simulink model "control_system"  (R2020b)
settings: Solver=FixedStepAuto  StartTime=0.0  StopTime=t_sim  FixedStep=Ts  RelTol=1e-2
values from neighbouring files (symbols this model uses):
  Hp = 10    [main_script.m]
  InitPosX = -2.4980e+03    (= -2498)    [main_script.m]
  InitPosY = -650.5503    [main_script.m]
  InitVelX = V0*cosd(InitYaw)    [main_script.m]
  InitVelY = V0*sind(InitYaw)    [main_script.m]
  InitYaw = 21    [main_script.m]
  lr = 1.592    [main_script.m]
  m = 1625    [main_script.m]
  Ts = 0.1    [main_script.m]
  V0 = 25    [main_script.m]
libraries: neural x856, simulink x1, autolibshared x1, drivingscenarioandsensors x1
(part 16 of 40)

== system control_system/50 30 1+2+3+14+15+19 ok curva sx1/Layer 3/Delays 1 ==
  "p{3}" : Inport  PortDimensions=30  SampleTime=0.1
      mask Display: e = 0.06;c1 = [120 230 180]/255;c2 = ([120 230 180]+0)/(256+128);c3 = ([120 230 180]+128)/(256+128);patch([0 1 1 0],[0 0 1 1],c1);patch([0 1 1 1-e 1-e 0+e],[0 0 1 1-e 0+e 0+e],c2);patch([0 0 1 1-e 0+e 0+e],[0 1 1 1-e 1-e 0+e],c3);plot([0 1 1 0 0],[0 0 1 1 0]);
  mux : Mux  Inputs=1
      mask Display: e = 0.06;c1 = [120 150 230]/255;c2 = ([120 150 230]+0)/383;c3 = ([120 150 230]+128)/383;patch([0 1 1 0],[0 0 1 1],c1);patch([0 1 1 1-e 1-e 0+e],[0 0 1 1-e 0+e 0+e],c2);patch([0 0 1 1-e 0+e 0+e],[0 1 1 1-e 1-e 0+e],c3);plot([0 1 1 0 0],[0 0 1 1 0]);disp('Mux')
  "pd{3,2}" : Outport
      mask Display: e = 0.06;c1 = [120 230 180]/255;c2 = ([120 230 180]+0)/(256+128);c3 = ([120 230 180]+128)/(256+128);patch([0 1 1 0],[0 0 1 1],c1);patch([0 1 1 1-e 1-e 0+e],[0 0 1 1-e 0+e 0+e],c2);patch([0 0 1 1-e 0+e 0+e],[0 1 1 1-e 1-e 0+e],c3);plot([0 1 1 0 0],[0 0 1 1 0]);
  wires:
  "p{3}"/1 -> mux/1
  mux/1 -> "pd{3,2}"/1

== system control_system/50 30 1+2+3+14+15+19 ok curva sx1/Layer 3/LW{3,2} ==
  "ad{3,2}" : Inport  PortDimensions=30  SampleTime=0.1
      mask Display: e = 0.06;c1 = [120 230 180]/255;c2 = ([120 230 180]+0)/(256+128);c3 = ([120 230 180]+128)/(256+128);patch([0 1 1 0],[0 0 1 1],c1);patch([0 1 1 1-e 1-e 0+e],[0 0 1 1-e 0+e 0+e],c2);patch([0 0 1 1-e 0+e 0+e],[0 1 1 1-e 1-e 0+e],c3);plot([0 1 1 0 0],[0 0 1 1 0]);
  "IW{3,2}(1,:)'" : Constant  Value=[0.2080002762427460016869673609107849188148975372314453125;-1.4701781861357201552920059839379973709583282470703125;0.5716293010951833952759670864907093346118927001953125;-2.091734276252824376030048370012082159519195556640625;-0.7232547294290245787351523176766932010650634765625;-0.7523031666304171860559790729894302785396575927734375;1.126506034122003452324634054093621671199798583984375;-0.7413157774186629467294551432132720947265625;4.0907595669557093032153716194443404674530029296875;-1.0909951695245292402347558891051448881626129150390625;1.546615937241918370403936933143995702266693115234375;-1.699729997229288525062429471290670335292816162109375;1.2641923780475516903010202440782450139522552490234375;-0.81857726118945828286399546414031647145748138427734375;-0.69223033284875568060812156545580364763736724853515625;1.3134722759902406341581126980599947273731231689453125;-0.09419836643332353542934498591421288438141345977783203125;1.3667404373136260442578304719063453376293182373046875;2.147315062483012848559837948414497077465057373046875;0.90329575973808406974541185263660736382007598876953125;-0.91494420597091874469697359018027782440185546875;0.11184734697806060499392089013781514950096607208251953125;2.137111480021808507245850705658085644245147705078125;0.8895719363186456174474869840196333825588226318359375;-1.4963687917207264543861811034730635583400726318359375;-1.31834627533638748531075179926119744777679443359375;-1.1370030127444248346790800496819429099559783935546875;-0.1538977545285384052053956338568241335451602935791015625;-0.29665226039340863994908659151406027376651763916015625;-1.43949303870013789463655484723858535289764404296875]
      mask Display: e = 0.06;c1 = [120 150 230]/255;c2 = ([120 150 230]+0)/383;c3 = ([120 150 230]+128)/383;patch([0 1 1 0],[0 0 1 1],c1);patch([0 1 1 1-e 1-e 0+e],[0 0 1 1-e 0+e 0+e],c2);patch([0 0 1 1-e 0+e 0+e],[0 1 1 1-e 1-e 0+e],c3);plot([0 1 1 0 0],[0 0 1 1 0]);disp('weights');
  "IW{3,2}(2,:)'" : Constant  Value=[0.46261036197923655066688297665677964687347412109375;-0.29462779673057870599706120628979988396167755126953125;0.370249630513741767590119025044259615242481231689453125;0.257922179946761975788405152343329973518848419189453125;0.73482180131654872834445768603472970426082611083984375;-0.411336645571016290556798367106239311397075653076171875;0.250506955966511568600907366999308578670024871826171875;-1.191518241329379890203199465759098529815673828125;0.5664750616390910042952100411639548838138580322265625;-0.10649560221090446920921834816908813081681728363037109375;0.03506241329652105831460318086101324297487735748291015625;0.250158860337789390460017102668643929064273834228515625;-0.2246735096171919021657004122971557080745697021484375;0.52214808664856804387710553783108480274677276611328125;-0.1996919451199098138882703779017901979386806488037109375;0.435200860233396602527733421084121800959110260009765625;-0.09546699455945463486106206119075068272650241851806640625;0.0862008075865288991845858390661305747926235198974609375;0.20696851436002983160022949959966354072093963623046875;0.09725975649991196181343156013099360279738903045654296875;0.208240927265578246174726473327609710395336151123046875;-0.0023995079288028756982209532822025721543468534946441650390625;0.141988662430395262692428559603285975754261016845703125;-0.1890063395171066584765640072873793542385101318359375;-0.160281565357498489987619905150495469570159912109375;0.065270878975224544404909465811215341091156005859375;-0.388208328639083444233648378940415568649768829345703125;0.16210529360622150107928973739035427570343017578125;-0.70678499559372076621599489953950978815555572509765625;0.032284673026462325229335448284473386593163013458251953125]
      mask Display: e = 0.06;c1 = [120 150 230]/255;c2 = ([120 150 230]+0)/383;c3 = ([120 150 230]+128)/383;patch([0 1 1 0],[0 0 1 1],c1);patch([0 1 1 1-e 1-e 0+e],[0 0 1 1-e 0+e 0+e],c2);patch([0 0 1 1-e 0+e 0+e],[0 1 1 1-e 1-e 0+e],c3);plot([0 1 1 0 0],[0 0 1 1 0]);disp('weights');
  Mux : Mux  Inputs=2
      mask Display: e = 0.06;c1 = [120 150 230]/255;c2 = ([120 150 230]+0)/383;c3 = ([120 150 230]+128)/383;patch([0 1 1 0],[0 0 1 1],c1);patch([0 1 1 1-e 1-e 0+e],[0 0 1 1-e 0+e 0+e],c2);patch([0 0 1 1-e 0+e 0+e],[0 1 1 1-e 1-e 0+e],c3);plot([0 1 1 0 0],[0 0 1 1 0]);disp('Mux');
  dotprod1 : neural/Weight Functions/dotprod
  dotprod2 : neural/Weight Functions/dotprod
  "lz{3,2}" : Outport
      mask Display: e = 0.06;c1 = [120 230 180]/255;c2 = ([120 230 180]+0)/(256+128);c3 = ([120 230 180]+128)/(256+128);patch([0 1 1 0],[0 0 1 1],c1);patch([0 1 1 1-e 1-e 0+e],[0 0 1 1-e 0+e 0+e],c2);patch([0 0 1 1-e 0+e 0+e],[0 1 1 1-e 1-e 0+e],c3);plot([0 1 1 0 0],[0 0 1 1 0]);
  wires:
  "IW{3,2}(1,:)'"/1 -> dotprod1/1
  "ad{3,2}"/1 -> dotprod1/2, dotprod2/2
  dotprod1/1 -> Mux/1
  "IW{3,2}(2,:)'"/1 -> dotprod2/1
  dotprod2/1 -> Mux/2
  Mux/1 -> "lz{3,2}"/1

== system control_system/50 30 1+2+3+14+15+19+22+23+24 curva dx 500m /Layer 1/Delays 1 ==
  "p{1}" : Inport  PortDimensions=18  SampleTime=0.1
      mask Display: e = 0.06;c1 = [120 230 180]/255;c2 = ([120 230 180]+0)/(256+128);c3 = ([120 230 180]+128)/(256+128);patch([0 1 1 0],[0 0 1 1],c1);patch([0 1 1 1-e 1-e 0+e],[0 0 1 1-e 0+e 0+e],c2);patch([0 0 1 1-e 0+e 0+e],[0 1 1 1-e 1-e 0+e],c3);plot([0 1 1 0 0],[0 0 1 1 0]);
  mux : Mux  Inputs=1
      mask Display: e = 0.06;c1 = [120 150 230]/255;c2 = ([120 150 230]+0)/383;c3 = ([120 150 230]+128)/383;patch([0 1 1 0],[0 0 1 1],c1);patch([0 1 1 1-e 1-e 0+e],[0 0 1 1-e 0+e 0+e],c2);patch([0 0 1 1-e 0+e 0+e],[0 1 1 1-e 1-e 0+e],c3);plot([0 1 1 0 0],[0 0 1 1 0]);disp('Mux')
  "pd{1,1}" : Outport
      mask Display: e = 0.06;c1 = [120 230 180]/255;c2 = ([120 230 180]+0)/(256+128);c3 = ([120 230 180]+128)/(256+128);patch([0 1 1 0],[0 0 1 1],c1);patch([0 1 1 1-e 1-e 0+e],[0 0 1 1-e 0+e 0+e],c2);patch([0 0 1 1-e 0+e 0+e],[0 1 1 1-e 1-e 0+e],c3);plot([0 1 1 0 0],[0 0 1 1 0]);
  wires:
  "p{1}"/1 -> mux/1
  mux/1 -> "pd{1,1}"/1
